simulink library "G2ELib_V1"  (R2020b)
settings: Solver=VariableStepAuto  StartTime=0.0  StopTime=10.0  RelTol=1e-3
undefined symbols (not defined in the file or in its folder): ee_sli_rtmsupport, Filter, Filter_I_ini, Filter_V_ini, gcbh, GFM, GFM_L2, GFM_R2, Parameters_Ib, Parameters_Sb, Parameters_Un_dc, q_filter_wf, References_Q, References_Theta_Eg0, simlt, sps_rtmsupport, Vdc_loop
libraries: powerlib x48, simulink_extras x11, eeTransforms x10, pid_lib x8, spsSourcesModel x3, powerlib_meascontrol x3, spsVIMeasurementModel x3, spsFirstOrderFilterModel x3, spsSynchronousMachineModel x3, eeGeneralControl x2, eePowerMeasurement x1, sps3phSaturableTransformerModel x1
(part 5 of 5)

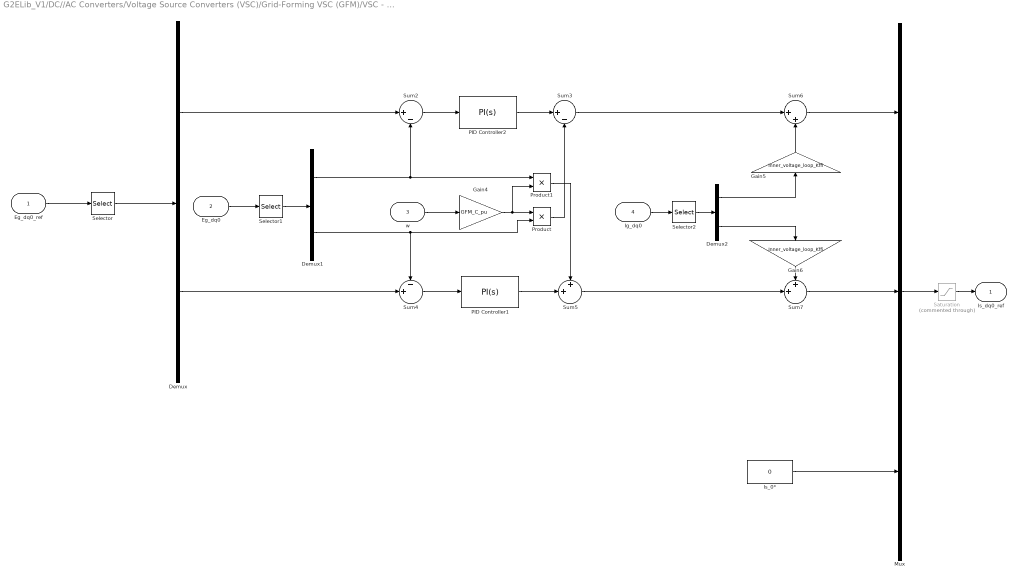
== system G2ELib_V1/DC//AC Converters/Voltage Source Converters (VSC)/Grid-Forming VSC (GFM)/VSC - GFM - Generic - Ideal/Voltage Loop ==
  Eg_dq0_ref : Inport
  Eg_dq0 : Inport  Port=2
  w : Inport  Port=3
  Ig_dq0 : Inport  Port=4
  Demux : Demux  Outputs=2
  Demux1 : Demux  Outputs=2
  Demux2 : Demux  Outputs=2
  Gain4 : Gain  Gain=GFM_C_pu
  Gain5 : Gain  Gain=Inner_voltage_loop_Kffi
  Gain6 : Gain  Gain=Inner_voltage_loop_Kffi
  Is_0* : Constant  Value=0
  Mux : Mux  Inputs=3
  PID Controller1 : pid_lib/PID Controller  Controller=PI  Form=Parallel  TimeDomain=Continuous-time  UseExternalTs=off  SampleTime=-1  IntegratorMethod=Forward Euler  FilterMethod=Forward Euler  ControllerParametersSource=internal  P=Inner_voltage_loop_Kp  I=Inner_voltage_loop_Ki  D=0  UseFilter=on  N=100  TunerSelectOption=Transfer Function Based (PID Tuner App)  InitialConditionSource=internal  InitialConditionForIntegrator=Inner_voltage_loop_Int_ini_q  InitialConditionForFilter=0  DifferentiatorICPrevScaledInput=0  ExternalReset=none  TrackingMode=off  Kt=1  LimitOutput=off  SatLimitsSource=internal  UpperSaturationLimit=inf  LowerSaturationLimit=-inf  LinearizeAsGain=on  AntiWindupMode=none  Kb=1  POutMin=[]  POutMax=[]  IOutMin=[]  IOutMax=[]  DOutMin=[]  DOutMax=[]  NOutMin=[]  NOutMax=[]  SumOutMin=[]  SumOutMax=[]  SaturationOutMin=[]  SaturationOutMax=[]  PParamMin=[]  PParamMax=[]  IParamMin=[]  IParamMax=[]  DParamMin=[]  DParamMax=[]  NParamMin=[]  NParamMax=[]  KbParamMin=[]  KbParamMax=[]  KtParamMin=[]  KtParamMax=[]  KbOutMin=[]  KbOutMax=[]  KtOutMin=[]  KtOutMax=[]  IntegratorOutMin=[]  IntegratorOutMax=[]  FilterOutMin=[]  FilterOutMax=[]  SumI1OutMin=[]  SumI1OutMax=[]  SumI2OutMin=[]  SumI2OutMax=[]  SumI3OutMin=[]  SumI3OutMax=[]  SumI4OutMin=[]  SumI4OutMax=[]  SumDOutMin=[]  SumDOutMax=[]  DifferentiatorOutMin=[]  DifferentiatorOutMax=[]  FilterDiffOutCoefMin=[]  FilterDiffOutCoefMax=[]  ReciprocalOutMin=[]  ReciprocalOutMax=[]  SumDenOutMin=[]  SumDenOutMax=[]  SumNumOutMin=[]  SumNumOutMax=[]  DivideOutMin=[]  DivideOutMax=[]  UdiffTsProdOutMin=[]  UdiffTsProdOutMax=[]  NTsProdOutMin=[]  NTsProdOutMax=[]  UintegralTsProdOutMin=[]  UintegralTsProdOutMax=[]  UngainTsProdOutMin=[]  UngainTsProdOutMax=[]  IntegratorContinuousStateAttributes=''  IntegratorStateMustResolveToSignalObject=off  IntegratorRTWStateStorageClass=Auto  FilterContinuousStateAttributes=''  FilterStateMustResolveToSignalObject=off  FilterRTWStateStorageClass=Auto  ParallelPVariant=InternalParameters  IdealPVariant=Disabled  IVariant=InternalParameters  DVariant=Disabled  IntegratorVariant=Continuous  SatVariant=Disabled  AWVariant=Passthrough  PCopyVariant=Disabled  TRVariant=Disabled  FdbkBlocksVariant=Forward  IdealPFdbkVariant=Disabled  SatFdbkVariant=Disabled  DerivativeFilterVariant=Disabled  NVariant=Disabled  NCopyVariant=Disabled_SignalSpec  FilterICVariant=Disabled  IntegratorICVariant=InternalICs  ExternalResetVariant=Disabled  TRSumVariant=Passthrough  SumFdbkVariant=Disabled  SumVariant=Sum_PI  TsampFilterVariant=InternalTs  TsampNgainVariant=Passthrough  TsampIntegralVariant=Passthrough  ExternalSaturationOutDataTypeStr=Inherit: Same as second input
  PID Controller2 : pid_lib/PID Controller  Controller=PI  Form=Parallel  TimeDomain=Continuous-time  UseExternalTs=off  SampleTime=-1  IntegratorMethod=Forward Euler  FilterMethod=Forward Euler  ControllerParametersSource=internal  P=Inner_voltage_loop_Kp  I=Inner_voltage_loop_Ki  D=0  UseFilter=on  N=100  TunerSelectOption=Transfer Function Based (PID Tuner App)  InitialConditionSource=internal  InitialConditionForIntegrator=Inner_voltage_loop_Int_ini_d  InitialConditionForFilter=0  DifferentiatorICPrevScaledInput=0  ExternalReset=none  TrackingMode=off  Kt=1  LimitOutput=off  SatLimitsSource=internal  UpperSaturationLimit=inf  LowerSaturationLimit=-inf  LinearizeAsGain=on  AntiWindupMode=none  Kb=1  POutMin=[]  POutMax=[]  IOutMin=[]  IOutMax=[]  DOutMin=[]  DOutMax=[]  NOutMin=[]  NOutMax=[]  SumOutMin=[]  SumOutMax=[]  SaturationOutMin=[]  SaturationOutMax=[]  PParamMin=[]  PParamMax=[]  IParamMin=[]  IParamMax=[]  DParamMin=[]  DParamMax=[]  NParamMin=[]  NParamMax=[]  KbParamMin=[]  KbParamMax=[]  KtParamMin=[]  KtParamMax=[]  KbOutMin=[]  KbOutMax=[]  KtOutMin=[]  KtOutMax=[]  IntegratorOutMin=[]  IntegratorOutMax=[]  FilterOutMin=[]  FilterOutMax=[]  SumI1OutMin=[]  SumI1OutMax=[]  SumI2OutMin=[]  SumI2OutMax=[]  SumI3OutMin=[]  SumI3OutMax=[]  SumI4OutMin=[]  SumI4OutMax=[]  SumDOutMin=[]  SumDOutMax=[]  DifferentiatorOutMin=[]  DifferentiatorOutMax=[]  FilterDiffOutCoefMin=[]  FilterDiffOutCoefMax=[]  ReciprocalOutMin=[]  ReciprocalOutMax=[]  SumDenOutMin=[]  SumDenOutMax=[]  SumNumOutMin=[]  SumNumOutMax=[]  DivideOutMin=[]  DivideOutMax=[]  UdiffTsProdOutMin=[]  UdiffTsProdOutMax=[]  NTsProdOutMin=[]  NTsProdOutMax=[]  UintegralTsProdOutMin=[]  UintegralTsProdOutMax=[]  UngainTsProdOutMin=[]  UngainTsProdOutMax=[]  IntegratorContinuousStateAttributes=''  IntegratorStateMustResolveToSignalObject=off  IntegratorRTWStateStorageClass=Auto  FilterContinuousStateAttributes=''  FilterStateMustResolveToSignalObject=off  FilterRTWStateStorageClass=Auto  ParallelPVariant=InternalParameters  IdealPVariant=Disabled  IVariant=InternalParameters  DVariant=Disabled  IntegratorVariant=Continuous  SatVariant=Disabled  AWVariant=Passthrough  PCopyVariant=Disabled  TRVariant=Disabled  FdbkBlocksVariant=Forward  IdealPFdbkVariant=Disabled  SatFdbkVariant=Disabled  DerivativeFilterVariant=Disabled  NVariant=Disabled  NCopyVariant=Disabled_SignalSpec  FilterICVariant=Disabled  IntegratorICVariant=InternalICs  ExternalResetVariant=Disabled  TRSumVariant=Passthrough  SumFdbkVariant=Disabled  SumVariant=Sum_PI  TsampFilterVariant=InternalTs  TsampNgainVariant=Passthrough  TsampIntegralVariant=Passthrough  ExternalSaturationOutDataTypeStr=Inherit: Same as second input
  Product : Product
  Product1 : Product
  Saturation : Saturate  Commented=through  UpperLimit=1  LowerLimit=-1
  Selector : Selector  InputPortWidth=3  IndexOptions=Index vector (dialog)  Indices=[1 2]  OutputSizes=1
  Selector1 : Selector  InputPortWidth=3  IndexOptions=Index vector (dialog)  Indices=[1 2]  OutputSizes=1
  Selector2 : Selector  InputPortWidth=3  IndexOptions=Index vector (dialog)  Indices=[1 2]  OutputSizes=1
  Sum2 : Sum  Inputs=|+-
  Sum3 : Sum  Inputs=|+-
  Sum4 : Sum  Inputs=-+|
  Sum5 : Sum  Inputs=++|
  Sum6 : Sum  Inputs=|++
  Sum7 : Sum  Inputs=++|
  Is_dq0_ref : Outport
  wires:
  Demux/2 -> Sum4/2
  Product1/1 -> Sum5/1
  Sum6/1 -> Mux/1
  Eg_dq0_ref/1 -> Selector/1
  Sum7/1 -> Mux/2
  Sum4/1 -> PID Controller1/1
  Sum5/1 -> Sum7/2
  Ig_dq0/1 -> Selector2/1
  Sum2/1 -> PID Controller2/1
  Gain6/1 -> Sum7/1
  Mux/1 -> Saturation/1
  Eg_dq0/1 -> Selector1/1
  Is_0*/1 -> Mux/3
  Selector2/1 -> Demux2/1
  w/1 -> Gain4/1
  Selector1/1 -> Demux1/1
  Product/1 -> Sum3/2
  Gain4/1 -> Product/1, Product1/2
  PID Controller1/1 -> Sum5/2
  Demux/1 -> Sum2/1
  Gain5/1 -> Sum6/2
  Sum3/1 -> Sum6/1
  Selector/1 -> Demux/1
  PID Controller2/1 -> Sum3/1
  Demux1/2 -> Product/2, Sum4/1
  Demux2/1 -> Gain5/1
  Demux2/2 -> Gain6/1
  Demux1/1 -> Product1/1, Sum2/2
  Saturation/1 -> Is_dq0_ref/1

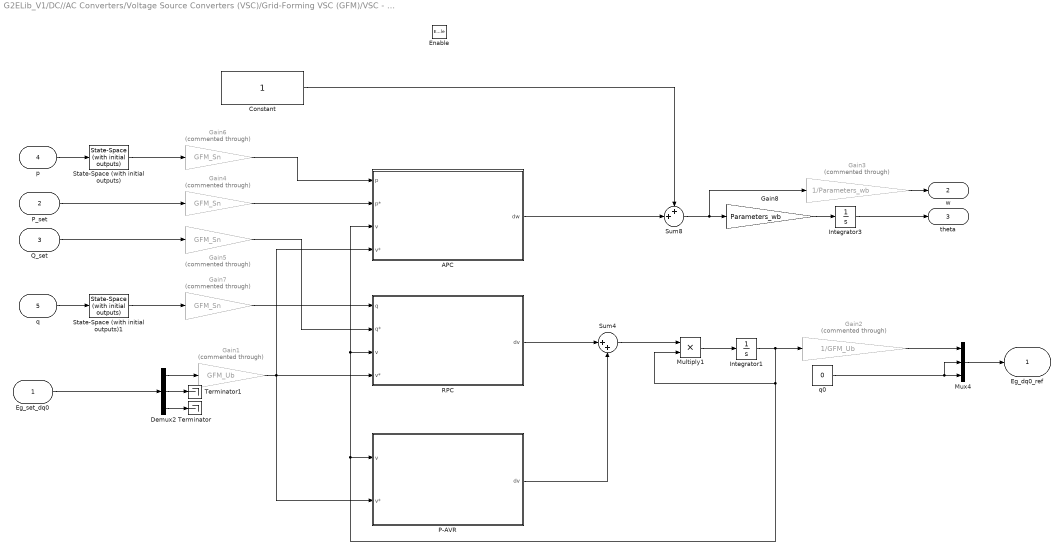
== system G2ELib_V1/DC//AC Converters/Voltage Source Converters (VSC)/Grid-Forming VSC (GFM)/VSC - GFM - Generic - Ideal/dVOC - P-f (PU)  ==
  Eg_set_dq0 : Inport
  P_set : Inport  Port=2
  Q_set : Inport  Port=3
  p : Inport  Port=4
  q : Inport  Port=5
  Enable : EnablePort
  APC : Subsystem
  Constant : Constant
  Demux2 : Demux  Outputs=3
  Gain1 : Gain  Commented=through  Gain=GFM_Ub
  Gain2 : Gain  Commented=through  Gain=1/GFM_Ub
  Gain3 : Gain  Commented=through  Gain=1/Parameters_wb
  Gain{4..7} (4 alike) : Gain  Commented=through  Gain=GFM_Sn
  Gain8 : Gain  Gain=Parameters_wb
  Integrator1 : Integrator  InitialCondition=GFM_Vref
  Integrator3 : Integrator  InitialCondition=GFM_Theta_Eg0
  Multiply1 : Product
  Mux4 : Mux  Inputs=3
  P-AVR : Subsystem
  RPC : Subsystem
  State-Space (with initial outputs) : simulink_extras/Additional Linear/State-Space (with initial outputs)  A=-q_filter_wf  B=1  C=q_filter_wf  D=0  U0=0  Y0=GFM_Pref
      settings: SourceProductBaseCode=SL
  State-Space (with initial outputs)1 : simulink_extras/Additional Linear/State-Space (with initial outputs)  A=-q_filter_wf  B=1  C=q_filter_wf  D=0  U0=0  Y0=GFM_Qref
      settings: SourceProductBaseCode=SL
  Sum4 : Sum  Inputs=|++
  Sum8 : Sum  Inputs=++|
  Terminator : Terminator
  Terminator1 : Terminator
  q0 : Constant  Value=0
  Eg_dq0_ref : Outport
  w : Outport  Port=2
  theta : Outport  Port=3
  wires:
  q/1 -> State-Space (with initial outputs)1/1
  p/1 -> State-Space (with initial outputs)/1
  APC/1(dw) -> Sum8/2
  Gain7/1 -> RPC/1(q)
  Gain6/1 -> APC/1(p)
  Gain3/1 -> w/1
  Gain2/1 -> Mux4/1
  Gain1/1 -> APC/4(v*), P-AVR/2(v*), RPC/4(v*)
  Q_set/1 -> Gain5/1
  P_set/1 -> Gain4/1
  Demux2/3 -> Terminator/1
  Multiply1/1 -> Integrator1/1
  Constant/1 -> Sum8/1
  Gain4/1 -> APC/2(p*)
  RPC/1(dv) -> Sum4/1
  P-AVR/1(dv) -> Sum4/2
  Sum4/1 -> Multiply1/1
  Integrator1/1 -> Multiply1/2, APC/3(v), RPC/3(v), P-AVR/1(v), Gain2/1
  Sum8/1 -> Gain8/1, Gain3/1
  q0/1 -> Mux4/3, Mux4/2
  Demux2/1 -> Gain1/1
  Gain5/1 -> RPC/2(q*)
  Integrator3/1 -> theta/1
  Mux4/1 -> Eg_dq0_ref/1
  Eg_set_dq0/1 -> Demux2/1
  Demux2/2 -> Terminator1/1
  State-Space (with initial outputs)/1 -> Gain6/1
  State-Space (with initial outputs)1/1 -> Gain7/1
  Gain8/1 -> Integrator3/1

== system G2ELib_V1/DC//AC Converters/Voltage Source Converters (VSC)/Grid-Forming VSC (GFM)/VSC - GFM - Generic - Ideal/Damping Resistor/Subsystem ==
  In1 : Inport
  Gain3 : Gain  Gain=Damping_resistor_W_RV
  Integrator1 : Integrator  InitialCondition=Damping_resistor_Int_ini
  Sum1 : Sum  Inputs=|+-
  Out1 : Outport
  wires:
  Gain3/1 -> Integrator1/1
  Sum1/1 -> Gain3/1
  In1/1 -> Sum1/1
  Integrator1/1 -> Out1/1, Sum1/2

== system G2ELib_V1/DC//AC Converters/Voltage Source Converters (VSC)/Grid-Forming VSC (GFM)/VSC - GFM - Generic - Ideal/VSM AVR (PU)/Park Transform2 ==
  abc : Inport
  theta : Inport  Port=2
  0 : Fcn  Expr=K1*(u(1) + u(2) + u(3))
  Gain1 : Gain  Gain=K2
  Mux2 : Mux  Inputs=2
  Mux3 : Mux  Inputs=3
  d : Fcn  Expr=sin(u(4)+Offset)*u(1) + sin(u(4)+Offset-2*pi/3)*u(2) + sin(u(4)+Offset+2*pi/3)*u(3)
  q : Fcn  Expr=cos(u(4)+Offset)*u(1) + cos(u(4)+Offset-2*pi/3)*u(2) + cos(u(4)+Offset+2*pi/3)*u(3)
  dq0 : Outport  VectorParamsAs1DForOutWhenUnconnected=off
  wires:
  0/1 -> Mux3/3
  Gain1/1 -> dq0/1
  Mux3/1 -> Gain1/1
  Mux2/1 -> 0/1, q/1, d/1
  theta/1 -> Mux2/2
  q/1 -> Mux3/2
  d/1 -> Mux3/1
  abc/1 -> Mux2/1

== system G2ELib_V1/DC//AC Converters/Voltage Source Converters (VSC)/Grid-Forming VSC (GFM)/VSC - GFM - Generic - Ideal/VSM AVR (PU)/emf_ calculation2 ==
  MfIf : Inport
  theta : Inport  Port=2
  w : Inport  Port=3
  Constant : Constant  Value=2*pi/3
  Constant1 : Constant  Value=4*pi/3
  Gain : Gain
  Mux : Mux  Inputs=3
  Product : Product  Inputs=3
  Product1 : Product  Inputs=3
  Product2 : Product  Inputs=3
  Sin : Trigonometry
  Sin1 : Trigonometry
  Sin2 : Trigonometry
  Sum : Sum  Inputs=|+-
  Sum1 : Sum  Inputs=|+-
  emf : Outport
  wires:
  Sum/1 -> Sin1/1
  Product1/1 -> Mux/2
  Sin/1 -> Product/1
  Constant/1 -> Sum/2
  Sin1/1 -> Product1/1
  Constant1/1 -> Sum1/2
  Sum1/1 -> Sin2/1
  Product/1 -> Mux/1
  Product2/1 -> Mux/3
  Sin2/1 -> Product2/1
  Gain/1 -> Product2/3, Product1/3, Product/3
  Mux/1 -> emf/1
  MfIf/1 -> Product2/2, Product1/2, Product/2
  w/1 -> Gain/1
  theta/1 -> Sum/1, Sum1/1, Sin/1

== system G2ELib_V1/DC//AC Converters/Voltage Source Converters (VSC)/Grid-Forming VSC (GFM)/VSC - GFM - Generic - Ideal/dVOC - P-f (PU) /APC ==
  p : Inport
  p* : Inport  Port=2
  v : Inport  Port=3
  v* : Inport  Port=4
  Constant : Constant  Value=1e-5
  Divide : Product  Inputs=*/
  Divide1 : Product  Inputs=*/
  Gain : Gain  Gain=dVOC_eta
  Square : Math  Operator=square  SignedPower=on  SaturateOnIntegerOverflow=on
  Square1 : Math  Operator=square  SignedPower=on  SaturateOnIntegerOverflow=on
  Sum : Sum  Inputs=|++
  Sum1 : Sum  Inputs=|-+
  dw : Outport  VectorParamsAs1DForOutWhenUnconnected=off
  wires:
  p*/1 -> Divide1/1
  p/1 -> Divide/1
  v/1 -> Square1/1
  Constant/1 -> Sum/1
  Sum/1 -> Divide/2
  v*/1 -> Square/1
  Square/1 -> Divide1/2
  Square1/1 -> Sum/2
  Divide/1 -> Sum1/1
  Divide1/1 -> Sum1/2
  Sum1/1 -> Gain/1
  Gain/1 -> dw/1

== system G2ELib_V1/DC//AC Converters/Voltage Source Converters (VSC)/Grid-Forming VSC (GFM)/VSC - GFM - Generic - Ideal/dVOC - P-f (PU) /P-AVR ==
  v : Inport
  v* : Inport  Port=2
  Divide : Product  Inputs=*/
  Gain : Gain  Gain=dVOC_eta*dVOC_alpha
  Square : Math  Operator=square  SignedPower=on  SaturateOnIntegerOverflow=on
  Square1 : Math  Operator=square  SignedPower=on  SaturateOnIntegerOverflow=on
  Sum1 : Sum  Inputs=|-+
  dv : Outport  VectorParamsAs1DForOutWhenUnconnected=off
  wires:
  v/1 -> Square1/1
  v*/1 -> Square/1
  Square/1 -> Sum1/2, Divide/2
  Sum1/1 -> Gain/1
  Square1/1 -> Sum1/1
  Gain/1 -> Divide/1
  Divide/1 -> dv/1

== system G2ELib_V1/DC//AC Converters/Voltage Source Converters (VSC)/Grid-Forming VSC (GFM)/VSC - GFM - Generic - Ideal/dVOC - P-f (PU) /RPC ==
  q : Inport
  q* : Inport  Port=2
  v : Inport  Port=3
  v* : Inport  Port=4
  Constant : Constant  Value=1e-5
  Divide : Product  Inputs=*/
  Divide1 : Product  Inputs=*/
  Gain : Gain  Gain=dVOC_eta
  Square : Math  Operator=square  SignedPower=on  SaturateOnIntegerOverflow=on
  Square1 : Math  Operator=square  SignedPower=on  SaturateOnIntegerOverflow=on
  Sum : Sum  Inputs=|++
  Sum1 : Sum  Inputs=|-+
  dv : Outport  VectorParamsAs1DForOutWhenUnconnected=off
  wires:
  q*/1 -> Divide1/1
  q/1 -> Divide/1
  Constant/1 -> Sum/1
  Sum/1 -> Divide/2
  v*/1 -> Square/1
  Square/1 -> Divide1/2
  Square1/1 -> Sum/2
  Divide/1 -> Sum1/1
  Divide1/1 -> Sum1/2
  Sum1/1 -> Gain/1
  Gain/1 -> dv/1
  v/1 -> Square1/1
